simulink model "KK101"  (R2023a)
settings: Solver=FixedStepAuto  StartTime=0.0  StopTime=inf  FixedStep=0.001  RelTol=1e-3  EnableMultiTasking=on
libraries: arduinolib x3
settings Model: ExtModeTrigDuration=2  Creator=Alireza  LastModifiedBy=Alireza
settings OptimizationCC: EnhancedBackFolding=on  PassReuseOutputArgsAs=Individual arguments  ZeroExternalMemoryAtStartup=off  ZeroInternalMemoryAtStartup=off  MaxStackSize=64  OptimizeBlockOrder=speed  DifferentSizesBufferReuse=on  OptimizationCustomize=off  EfficientTunableParamExpr=on
settings DebuggingCC: ParameterTunabilityLossMsg=error
settings HardwareCC: ProdBitPerInt=16  ProdBitPerPointer=16  ProdBitPerSizeT=16  ProdBitPerPtrDiffT=16  ProdLargestAtomicFloat=None  ProdWordSize=8  ProdHWDeviceType=Atmel->AVR
settings SFSimCC: MATLABDynamicMemAlloc=off  SimTargetLang=C++  GPUAcceleration=on  SimDLTargetLibrary=cudnn
settings RTWCC: Description=Embedded Coder  SystemTargetFile=ert.tlc  HardwareBoard=Arduino Uno  TemplateMakefile=ert_default_tmf  Toolchain=Arduino AVR  BuildConfiguration=Faster Runs
settings CodeAppCC: ForceParamTrailComments=on  IgnoreCustomStorageClasses=off  OperatorAnnotations=on  SimulinkDataObjDesc=on  SFDataObjDesc=on  InsertBlockDesc=on
settings ERTTargetCC: SupportContinuousTime=on  SupportVariableSizeSignals=on  ExtModeTransport=3  ExtModeStaticAlloc=on  ExtModeAutomaticAllocSize=off  ExtModeStaticAllocSize=250  ExtModeMexFile=ext_xcp  ExtModeIntrfLevel=Level2 - Open

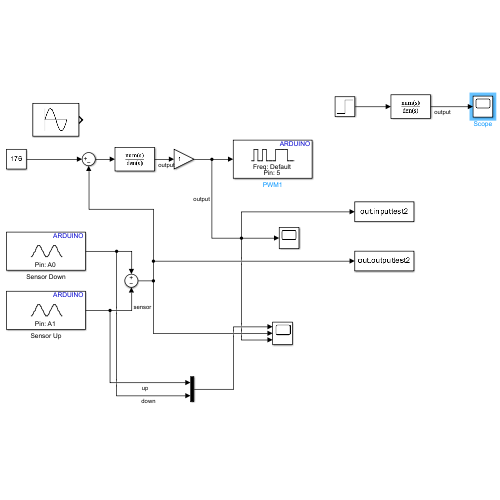
[thumbnail: Simulink's stored preview of the top-level diagram]
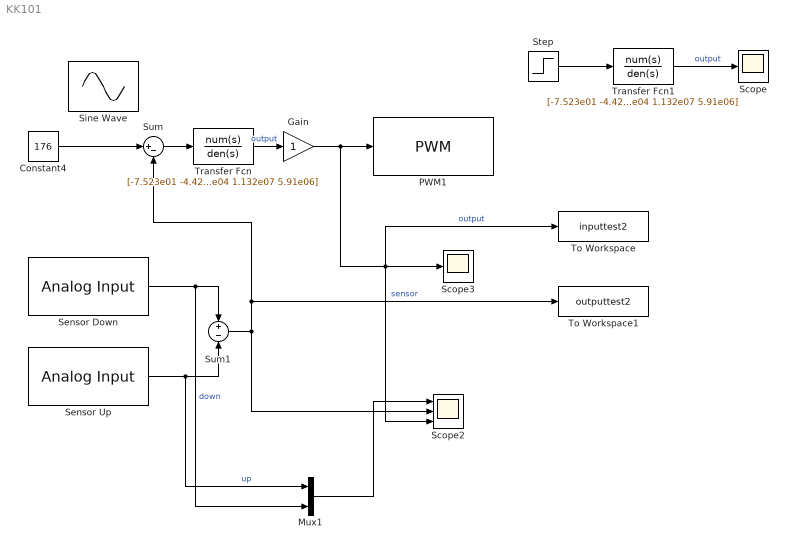
== system KK101 ==
  Constant4 : Constant  Value=176
  Gain : Gain
  Mux1 : Mux  Inputs=2
  PWM1 : arduinolib/PWM  pinNumber=5  frequencyType=Default  desiredFrequency=490.2  achievableFrequency=490.2
  Scope : Scope
  Scope2 : Scope  NumInputPorts=3
  Scope3 : Scope
  Sensor Down : arduinolib/Analog Input  pinNumber=0  ReadResultsOnly=off  ConversionTriggerSource=Software  ExternalTriggerType=uint32( 0 )  OutputDataType=uint16  EnableConversionCompleteNotify=off  EnableOuputStatus=off  SampleTime=0.001  blockPlatform=arduino
  Sensor Up : arduinolib/Analog Input  pinNumber=1  ReadResultsOnly=off  ConversionTriggerSource=Software  ExternalTriggerType=uint32( 0 )  OutputDataType=uint16  EnableConversionCompleteNotify=off  EnableOuputStatus=off  SampleTime=0.001  blockPlatform=arduino
  Sine Wave : Sin  Amplitude=0  Bias=155  Frequency=4  SampleTime=0
  Step : Step  SampleTime=0
  Sum : Sum  Inputs=|+-
  Sum1 : Sum  Inputs=+|-
  To Workspace : ToWorkspace  VariableName=inputtest2  SampleTime=0.001
      settings: Save2DSignal=2-D array (concatenate along first dimension)
  To Workspace1 : ToWorkspace  VariableName=outputtest2  SampleTime=0.001
      settings: Save2DSignal=2-D array (concatenate along first dimension)
  Transfer Fcn : TransferFcn  Numerator=[-7.523e01 -4.425e03 -1.093e04 -8.398e03]  Denominator=[1 1.959e04 1.132e07 5.91e06]
  Transfer Fcn1 : TransferFcn  Numerator=[-7.523e01 -4.425e03 -1.093e04 -8.398e03]  Denominator=[1 1.959e04 1.132e07 5.91e06]
  wires:
  Sensor Down/1 -> Mux1/2, Sum1/1  "down"
  Sensor Up/1 -> Mux1/1, Sum1/2  "up"
  Sum1/1 -> Scope2/2, To Workspace1/1, Sum/2  "sensor"
  Mux1/1 -> Scope2/1
  Sum/1 -> Transfer Fcn/1
  Gain/1 -> To Workspace/1, Scope2/3, Scope3/1, PWM1/1  "output"
  Constant4/1 -> Sum/1
  Transfer Fcn/1 -> Gain/1  "output"
  Step/1 -> Transfer Fcn1/1
  Transfer Fcn1/1 -> Scope/1  "output"
